simulink model "h01_MdeMgmt"  (R2024a)
settings: Solver=FixedStepDiscrete  StartTime=0.0  StopTime=mSim.dTime  FixedStep=mSim.dTime  MaxStep=0.0001  RelTol=0.0001
undefined symbols (not defined in the file): H01MDE, H01TRT
settings Model: Creator=admin  LastModifiedBy=admin
settings SolverCC: MaxConsecutiveZCs=10000  ZeroCrossAlgorithm=Adaptive  AlgebraicLoopSolver=TrustRegion
settings DataIOCC: SaveOutput=off  DSMLogging=off  InspectSignalLogs=on  SaveTime=off  SignalLoggingName=logsout_Validator
settings OptimizationCC: BlockReduction=off  DefaultParameterBehavior=Inlined  UseDivisionForNetSlopeComputation=UseDivisionForReciprocalsOfIntegersOnly  GainParamInheritBuiltInType=on  UseFloatMulNetSlope=on  DefaultUnderspecifiedDataType=single  InlineInvariantSignals=on  BitwiseOrLogicalOp=Logical operator  PassReuseOutputArgsAs=Individual arguments  EfficientFloat2IntCast=on  LifeSpan=Inf  OptimizeBlockOrder=speed  DifferentSizesBufferReuse=on  EfficientTunableParamExpr=on
settings DebuggingCC: SignalInfNanChecking=error  SignalRangeChecking=error  ReadBeforeWriteMsg=EnableAllAsError  WriteAfterWriteMsg=EnableAllAsError  WriteAfterReadMsg=EnableAllAsError  AlgebraicLoopMsg=error  ArtificialAlgebraicLoopMsg=error  SaveWithDisabledLinksMsg=error  SaveWithParameterizedLinksMsg=error  BlockPriorityViolationMsg=error  SolverPrmCheckMsg=error  InheritedTsInSrcMsg=error  SingleTaskRateTransMsg=error  TasksWithSamePriorityMsg=error  SigSpecEnsureSampleTimeMsg=error  CheckMatrixSingularityMsg=error  IntegerOverflowMsg=error  ParameterUnderflowMsg=error  ParameterPrecisionLossMsg=error  ParameterTunabilityLossMsg=error  UnderSpecifiedDataTypeMsg=error  UnnecessaryDatatypeConvMsg=warning  VectorMatrixConversionMsg=error  SignalLabelMismatchMsg=error  UnconnectedInputMsg=error  UnconnectedOutputMsg=error  UnconnectedLineMsg=error  SFcnCompatibilityMsg=error  UniqueDataStoreMsg=error  BusObjectLabelMismatch=error  RootOutportRequireBusObject=error  AssertControl=DisableAll  ModelReferenceIOMismatchMessage=error  UnknownTsInhSupMsg=error  ModelReferenceDataLoggingMessage=error  ModelReferenceSymbolNameMessage=none  StateNameClashWarn=warning  StrictBusMsg=ErrorOnBusTreatedAsVector  NonBusSignalsTreatedAsBus=error  SFInvalidInputDataAccessInChartInitDiag=error  SFTransitionOutsideNaturalParentDiag=error  SFUnreachableExecutionPathDiag=error  SFUndirectedBroadcastEventsDiag=error  SFTransitionActionBeforeConditionDiag=error  SFTemporalDelaySmallerThanSampleTimeDiag=error  SFSelfTransitionDiag=error  SFExecutionAtInitializationDiag=error  IntegerSaturationMsg=error  UnitsInconsistencyMsg=none  VariantConditionMismatch=error
settings HardwareCC: ProdBitPerPointer=32  ProdBitPerSizeT=32  ProdBitPerPtrDiffT=32  ProdLargestAtomicFloat=None  ProdWordSize=32  ProdLongLongMode=on  ProdHWDeviceType=Renesas->RH850
settings ModelReferenceCC: EnableRefExpFcnMdlSchedulingChecks=on  ModelReferenceNumInstancesAllowed=Single
settings SFSimCC: SimUseLocalCustomCode=off  CompileTimeRecursionLimit=0  EnableRuntimeRecursion=off  MATLABDynamicMemAlloc=off  CustomCodeUndefinedFunction=UseInterfaceOnly
settings RTWCC: Description=Embedded Coder  SystemTargetFile=ert.tlc  GenCodeOnly=on  TemplateMakefile=ert_default_tmf  GenerateReport=on  RTWUseLocalCustomCode=off  BuildConfiguration=Faster Runs  IncludeHyperlinkInReport=on  LaunchReport=on  GenerateTraceInfo=on  GenerateTraceReport=on  GenerateTraceReportSl=on  GenerateTraceReportSf=on  GenerateWebview=on  GenerateCodeMetricsReport=on  GenerateCodeReplacementReport=on  GPUComputeCapability=3.5  DLArmComputeVersion=19.05
settings RTWCC: CustomInclude=|
  | D:\1_Code\1_DWDC_CSPLUS_RH850\EX_EcompM24aBswR22\DWDCC_SW45CCLV_E2GHSM24A\TEMP
  | D:\1_Code\1_DWDC_CSPLUS_RH850\EX_EcompM24aBswR22\DWDCC_SW45CCLV_E2GHSM24A\ASW\eCompMbdCodeRlt\b01_OSnScheduler_ert_rtw
  | D:\1_Code\1_DWDC_CSPLUS_RH850\EX_EcompM24aBswR22\DWDCC_SW45CCLV_E2GHSM24A\ASW\eCompMbdCodeRlt\c01_MainAdc_ert_rtw
  | D:\1_Code\1_DWDC_CSPLUS_RH850\EX_EcompM24aBswR22\DWDCC_SW45CCLV_E2GHSM24A\ASW\eCompMbdCodeRlt\c02_SubAdc_ert_rtw
  | D:\1_Code\1_DWDC_CSPLUS_RH850\EX_EcompM24aBswR22\DWDCC_SW45CCLV_E2GHSM24A\ASW\eCompMbdCodeRlt\d01_Diaglnteg_ert_rtw
  | D:\1_Code\1_DWDC_CSPLUS_RH850\EX_EcompM24aBswR22\DWDCC_SW45CCLV_E2GHSM24A\ASW\eCompMbdCodeRlt\e01_MtrCtrl_VarGain_ert_rtw
  | D:\1_Code\1_DWDC_CSPLUS_RH850\EX_EcompM24aBswR22\DWDCC_SW45CCLV_E2GHSM24A\ASW\eCompMbdCodeRlt\e02_MtrCtrl_EstPst_ert_rtw
  | D:\1_Code\1_DWDC_CSPLUS_RH850\EX_EcompM24aBswR22\DWDCC_SW45CCLV_E2GHSM24A\ASW\eCompMbdCodeRlt\e03_MtrCtrl_MtrCtrl_ert_rtw
  | D:\1_Code\1_DWDC_CSPLUS_RH850\EX_EcompM24aBswR22\DWDCC_SW45CCLV_E2GHSM24A\ASW\eCompMbdCodeRlt\e04_MtrCtrl_PwmSet_ert_rtw
  | D:\1_Code\1_DWDC_CSPLUS_RH850\EX_EcompM24aBswR22\DWDCC_SW45CCLV_E2GHSM24A\ASW\eCompMbdCodeRlt\f01_CommRx1_ert_rtw
  | D:\1_Code\1_DWDC_CSPLUS_RH850\EX_EcompM24aBswR22\DWDCC_SW45CCLV_E2GHSM24A\ASW\eCompMbdCodeRlt\g01_CommTxDataSet1_ert_rtw
  | D:\1_Code\1_DWDC_CSPLUS_RH850\EX_EcompM24aBswR22\DWDCC_SW45CCLV_E2GHSM24A\ASW\eCompMbdCodeRlt\g02_CommTxDataSet2_ert_rtw
  | D:\1_Code\1_DWDC_CSPLUS_RH850\EX_EcompM24aBswR22\DWDCC_SW45CCLV_E2GHSM24A\ASW\eCompMbdCodeRlt\g03_CommTx_ert_rtw
  | D:\1_Code\1_DWDC_CSPLUS_RH850\EX_EcompM24aBswR22\DWDCC_SW45CCLV_E2GHSM24A\ASW\eCompMbdCodeRlt\h01_MdeMgmt_ert_rtw
  | D:\1_Code\1_DWDC_CSPLUS_RH850\EX_EcompM24aBswR22\DWDCC_SW45CCLV_E2GHSM24A\ASW\eCompMbdCodeRlt\i01_Dem_ert_rtw
  | D:\1_Code\1_DWDC_CSPLUS_RH850\EX_EcompM24aBswR22\DWDCC_SW45CCLV_E2GHSM24A\ASW\eCompMbdCodeRlt\j01_McuInit_ert_rtw
  | D:\1_Code\1_DWDC_CSPLUS_RH850\EX_EcompM24aBswR22\DWDCC_SW45CCLV_E2GHSM24A\ASW\eCompMbdCodeRlt\k01_NvM_ert_rtw
  | D:\1_Code\1_DWDC_CSPLUS_RH850\EX_EcompM24aBswR22\DWDCC_SW45CCLV_E2GHSM24A\ASW\eCompMbdCodeRlt\slprj\ert\_sharedutils
settings RTWCC: CustomInitializer=|
  | /* MISRA-C Dummy Code */
  | // H01STMDE.uDummy = 0U;
settings CodeAppCC: ForceParamTrailComments=on  IgnoreCustomStorageClasses=off  MATLABFcnDesc=on  MangleLength=4  CustomSymbolStrGlobalVar=GvH01$N$M  CustomSymbolStrType=StrH01$N$M  CustomSymbolStrFcn=$N$M$F  CustomSymbolStrMacro=$N$M  DefineNamingRule=UpperCase  ParamNamingRule=UpperCase  SimulinkBlockComments=off  EnableCustomComments=on  ReqsInCode=on
settings ERTTargetCC: UtilityFuncGeneration=Shared location  MultiwordLength=2048  IncludeMdlTerminateFcn=off  CombineSignalStateStructs=on  SuppressErrorStatus=on  SupportAbsoluteTime=off  SupportNonFinite=off  ParenthesesLevel=Maximum  CastingMode=Standards  GenerateSharedConstants=off  InlinedParameterPlacement=NonHierarchical  ERTSrcFileBannerTemplate=t_code_template.cgt  ERTHdrFileBannerTemplate=t_code_template.cgt  ERTDataSrcFileTemplate=t_code_template.cgt  ERTDataHdrFileTemplate=t_code_template.cgt  ERTCustomFileTemplate=example_file_process.tlc  ERTFilePackagingFormat=CompactWithDataFile  PreserveExpressionOrder=on  SuppressUnreachableDefaultCases=off  EnableSignedLeftShifts=off  EnableSignedRightShifts=off  IndentStyle=Allman  IndentSize=4
settings ConfigComp: CovSaveName=coveragedata  CovMetricSettings=we  CovEnableCumulative=off  CovSaveCumulativeToWorkspaceVar=on  CovSaveSingleToWorkspaceVar=on  CovOutputDir=sldv_output/$ModelName$\sldv_covoutput  PSModelRefIgnoreList=[]  PSEnableModelRefIgnoreList=off  PSModelRefMinMaxVerif=CheckAndConstrain  PSAutoStubLUT=on  DVTestSuiteOptimization=CombinedObjectives (Nonlinear Extended)  DVRebuildModelRepresentation=Always
settings SimscapeCC: SimscapeNormalizeSystem=off

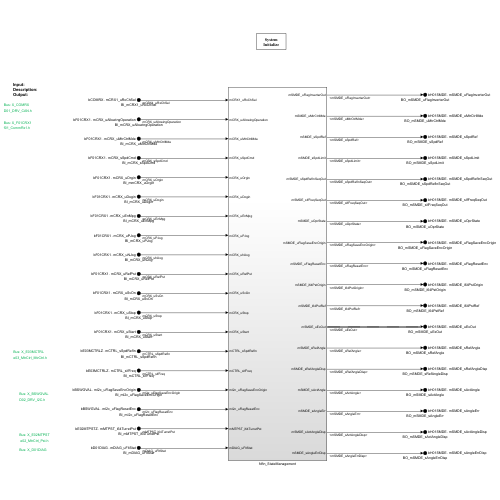
[thumbnail: Simulink's stored preview of the top-level diagram]
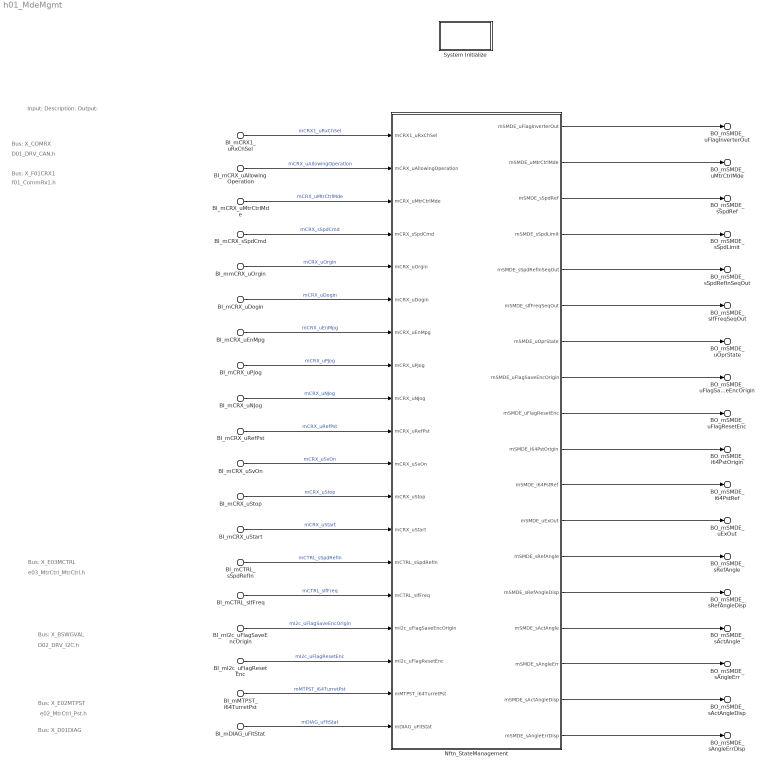
== system h01_MdeMgmt ==
  note: Bus: X_COMRX
  note: Bus: X_E03MCTRL
  note: e03_MtrCtrl_MtrCtrl.h
  note: D01_DRV_CAN.h
  note: Bus: X_BSWGVAL
  note: Bus: X_F01CRX1
  note: Input:
      | Description:
      | Output:
  note: Bus: X_E02MTPST
  note: e02_MtrCtrl_Pst.h
  note: D02_DRV_I2C.h
  note: f01_CommRx1.h
  note: Bus: X_D01DIAG
  BI_mCRX1_uRxChSel : Inport  Description=■ 설명: 운전 모드 설정 (0: I/O, 1: 통신)  PortName=bCOMRX  Element=mCRX1_uRxChSel
  BI_mCRX_uAllowingOperation : Inport  Description=■ 설명: 통신 모드 구동 신호 (0: 미구동, 1: 구동)  Port=2  PortName=bF01CRX1  Element=mCRX_uAllowingOperation
  BI_mCRX_uMtrCtrlMde : Inport  Description=■ 설명: 모터 구동 모드 (1_VF/2_V/4_CURR/8_TQ/16_SPD/32_PST/64_VALIGN/128_ALIGN/256_IF)  Port=2  PortName=bF01CRX1  Element=mCRX_uMtrCtrlMde
  BI_mCRX_uSvOn : Inport  Description=■ 설명: Digital Input Signal (서보 모터의 구동 신호, 0: 정지, 1: 구동)  Port=2  PortName=bF01CRX1  Element=mCRX_uSvOn
  BI_mCRX_uStart : Inport  Description=■ 설명: Digital Input Signal (구동 시작 신호, 상승 엣지 후 100msec 이상 검출 시 활성화)  Port=2  PortName=bF01CRX1  Element=mCRX_uStart
  BI_mCRX_uRefPst : Inport  Description=■ 설명: Digital Input Signal (위치 데이터 입력 신호 6Bit Binary Code)  Port=2  PortName=bF01CRX1  Element=mCRX_uRefPst
  BI_mCRX_uStop : Inport  Description=■ 설명: Digital Input Signal (동작 완료 신호)  Port=2  PortName=bF01CRX1  Element=mCRX_uStop
  BI_mmCRX_uOrgin : Inport  Description=■ 설명: Digital Input Signal (원점 설정 신호, 0: NA, 1: 원점 설정 활성화)  Port=2  PortName=bF01CRX1  Element=mCRX_uOrgin
  BI_mCRX_uDogin : Inport  Description=■ 설명: Digital Input Signal (원점 설정 초기화 신호, 0: NA, 1: 원점 초기화 활성화)  Port=2  PortName=bF01CRX1  Element=mCRX_uDogin
  BI_mCRX_uPJog : Inport  Description=■ 설명: Digital Input Signal (Manual CCW 구동 신호)  Port=2  PortName=bF01CRX1  Element=mCRX_uPJog
  BI_mCRX_uNJog : Inport  Description=■ 설명: Digital Input Signal (Manual CW 구동 신호)  Port=2  PortName=bF01CRX1  Element=mCRX_uNJog
  BI_mCRX_uEnMpg : Inport  Description=■ 설명: Digital Input Signal (미세 또는 단위 운전 설정, 0: 단위 운전, 1: 미세 운전)  Port=2  PortName=bF01CRX1  Element=mCRX_uEnMpg
  BI_mCRX_sSpdCmd : Inport  Description=■ 설명: 통신 모드 속도 지령  Port=2  PortName=bF01CRX1  Element=mCRX_sSpdCmd
  BI_mCTRL_sIfFreq : Inport  Description=■ 설명: IF Control Frequency  Port=3  PortName=bE03MCTRLZ  Element=mCTRL_sIfFreq
  BI_mCTRL_sSpdRefIn : Inport  Description=■ 설명: 속도 Slop 지령  Port=3  PortName=bE03MCTRLZ  Element=mCTRL_sSpdRefIn
  BI_mI2c_uFlagSaveEncOrigin : Inport  Description=■ 설명: 엔코더 원점 저장 활성화 신호  Port=4  PortName=bBSWGVAL  Element=mI2c_uFlagSaveEncOrigin
  BI_mI2c_uFlagResetEnc : Inport  Description=■ 설명: 엔코더 멀티턴 리셋 활성화 신호  Port=4  PortName=bBSWGVAL  Element=mI2c_uFlagResetEnc
  BI_mMTPST_i64TurretPst : Inport  Description=■ 설명: Turret Position  Port=5  PortName=bE02MTPSTZ  Element=mMTPST_i64TurretPst
  BI_mDIAG_uFltStat : Inport  Description=■ 설명: 고장 신호 대표 값  Port=6  PortName=bD01DIAG  Element=mDIAG_uFltStat
  Nftn_StateManagement : Subsystem
  System Initialize : Subsystem  mask(System Initialize){ShowInLibBrowser=0}
      mask prompts: ShowInLibBrowser "Simulink:masks:CustCodeMaskParam1_MP"
      settings: CopyFcn=cccopyfcn(gcb)  OpenFcn=ccopenfcn('System Initialize Function')
      mask Help: eval('feval(''rtwprivate'',''rtwhelpview'',''rtw_sys_initialize_block'')');
      mask DialogControl ShowInLibBrowser Prompt: 마스크 파라미터 1:
      mask Display: disp('System\nInitialize');
  BO_mSMDE_uFlagInverterOut : Outport  Description=■ 설명: Allow Operation 신호 (0: 구정 정지, 1: 구동)  PortName=bH01SMDE  Element=mSMDE_uFlagInverterOut
  BO_mSMDE_sSpdRefInSeqOut : Outport  Description=■ 설명: Speed Slop 제어를 위한 이전 지령 속도  PortName=bH01SMDE  Element=mSMDE_sSpdRefInSeqOut
  BO_mSMDE_sSpdLimit : Outport  Description=■ 설명: 속도 제한값  PortName=bH01SMDE  Element=mSMDE_sSpdLimit
  BO_mSMDE_sSpdRef : Outport  Description=■ 설명: 속도 지령  PortName=bH01SMDE  Element=mSMDE_sSpdRef
  BO_mSMDE_sIfFreqSeqOut : Outport  Description=■ 설명: 모터 구동 모드 (0_IO/1_VF/2_V/4_CURR/8_TQ/16_SPD/32_PST/64_VALIGN/128_ALIGN/256_IF)  PortName=bH01SMDE  Element=mSMDE_sIfFreqSeqOut
  BO_mSMDE_uMtrCtrlMde : Outport  Description=■ 설명: 운영 모드 (모터 구동 모드)  PortName=bH01SMDE  Element=mSMDE_uMtrCtrlMde
  BO_mSMDE_uOprState : Outport  Description=■ 설명: 운영 모드 (1H : Standby / 2H : JOG / 4H : MPG_JOG / 8H: Operating / 16H : Wait / 32H: Origin)  PortName=bH01SMDE  Element=mSMDE_uOprState
  BO_mSMDE_uFlagSaveEncOrigin : Outport  Description=■ 설명: 엔코더 원점 저장 활성화 신호  PortName=bH01SMDE  Element=mSMDE_uFlagSaveEncOrigin
  BO_mSMDE_uFlagResetEnc : Outport  Description=■ 설명: 엔코더 멀티턴 리셋 활성화 신호  PortName=bH01SMDE  Element=mSMDE_uFlagResetEnc
  BO_mSMDE_i64PstOrigin : Outport  Description=■ 설명: Encoder 원점 정보  PortName=bH01SMDE  Element=mSMDE_i64PstOrigin
  BO_mSMDE_i64PstRef : Outport  Description=■ 설명: Position Reference  PortName=bH01SMDE  Element=mSMDE_i64PstRef
  BO_mSMDE_sRefAngleDisp : Outport  Description=■ 설명: 터렛 지령 위치 모니터 값  PortName=bH01SMDE  Element=mSMDE_sRefAngleDisp
  BO_mSMDE_sActAngleDisp : Outport  Description=■ 설명: 터렛 지령 위치 모니터 값  PortName=bH01SMDE  Element=mSMDE_sActAngleDisp
  BO_mSMDE_sAngleErrDisp : Outport  Description="■ 설명: 터렛 현재 위치  오차 모니터 값"  PortName=bH01SMDE  Element=mSMDE_sAngleErrDisp
  BO_mSMDE_sRefAngle : Outport  Description=■ 설명: 터렛 지령 위치  PortName=bH01SMDE  Element=mSMDE_sRefAngle
  BO_mSMDE_sActAngle : Outport  Description=■ 설명: 터렛 현재 위치  PortName=bH01SMDE  Element=mSMDE_sActAngle
  BO_mSMDE_sAngleErr : Outport  Description=■ 설명: 터렛 위치 오차  PortName=bH01SMDE  Element=mSMDE_sAngleErr
  BO_mSMDE_uExOut : Outport  PortName=bH01SMDE  Element=mSMDE_uExOut
  wires:
  Nftn_StateManagement/8(mSMDE_uFlagSaveEncOrigin) -> BO_mSMDE_uFlagSaveEncOrigin/1
  Nftn_StateManagement/14(mSMDE_sRefAngleDisp) -> BO_mSMDE_sRefAngleDisp/1
  Nftn_StateManagement/17(mSMDE_sActAngleDisp) -> BO_mSMDE_sActAngleDisp/1
  BI_mCTRL_sIfFreq/1 -> Nftn_StateManagement/15(mCTRL_sIfFreq)  "mCTRL_sIfFreq"
  BI_mCRX_uMtrCtrlMde/1 -> Nftn_StateManagement/3(mCRX_uMtrCtrlMde)  "mCRX_uMtrCtrlMde"
  Nftn_StateManagement/18(mSMDE_sAngleErrDisp) -> BO_mSMDE_sAngleErrDisp/1
  BI_mCRX_uStop/1 -> Nftn_StateManagement/12(mCRX_uStop)  "mCRX_uStop"
  BI_mCRX_uSvOn/1 -> Nftn_StateManagement/11(mCRX_uSvOn)  "mCRX_uSvOn"
  BI_mCRX_uRefPst/1 -> Nftn_StateManagement/10(mCRX_uRefPst)  "mCRX_uRefPst"
  Nftn_StateManagement/7(mSMDE_uOprState) -> BO_mSMDE_uOprState/1
  Nftn_StateManagement/6(mSMDE_sIfFreqSeqOut) -> BO_mSMDE_sIfFreqSeqOut/1
  BI_mCRX_uNJog/1 -> Nftn_StateManagement/9(mCRX_uNJog)  "mCRX_uNJog"
  BI_mCRX_uAllowingOperation/1 -> Nftn_StateManagement/2(mCRX_uAllowingOperation)  "mCRX_uAllowingOperation"
  Nftn_StateManagement/16(mSMDE_sAngleErr) -> BO_mSMDE_sAngleErr/1
  BI_mCRX1_uRxChSel/1 -> Nftn_StateManagement/1(mCRX1_uRxChSel)  "mCRX1_uRxChSel"
  BI_mCRX_uStart/1 -> Nftn_StateManagement/13(mCRX_uStart)  "mCRX_uStart"
  Nftn_StateManagement/13(mSMDE_sRefAngle) -> BO_mSMDE_sRefAngle/1
  Nftn_StateManagement/15(mSMDE_sActAngle) -> BO_mSMDE_sActAngle/1
  BI_mCRX_sSpdCmd/1 -> Nftn_StateManagement/4(mCRX_sSpdCmd)  "mCRX_sSpdCmd"
  Nftn_StateManagement/1(mSMDE_uFlagInverterOut) -> BO_mSMDE_uFlagInverterOut/1
  BI_mCRX_uPJog/1 -> Nftn_StateManagement/8(mCRX_uPJog)  "mCRX_uPJog"
  Nftn_StateManagement/3(mSMDE_sSpdRef) -> BO_mSMDE_sSpdRef/1
  Nftn_StateManagement/5(mSMDE_sSpdRefInSeqOut) -> BO_mSMDE_sSpdRefInSeqOut/1
  BI_mI2c_uFlagResetEnc/1 -> Nftn_StateManagement/17(mI2c_uFlagResetEnc)  "mI2c_uFlagResetEnc"
  Nftn_StateManagement/9(mSMDE_uFlagResetEnc) -> BO_mSMDE_uFlagResetEnc/1
  Nftn_StateManagement/11(mSMDE_i64PstRef) -> BO_mSMDE_i64PstRef/1
  Nftn_StateManagement/10(mSMDE_i64PstOrigin) -> BO_mSMDE_i64PstOrigin/1
  BI_mCTRL_sSpdRefIn/1 -> Nftn_StateManagement/14(mCTRL_sSpdRefIn)  "mCTRL_sSpdRefIn"
  BI_mmCRX_uOrgin/1 -> Nftn_StateManagement/5(mCRX_uOrgin)  "mCRX_uOrgin"
  BI_mMTPST_i64TurretPst/1 -> Nftn_StateManagement/18(mMTPST_i64TurretPst)  "mMTPST_i64TurretPst"
  BI_mDIAG_uFltStat/1 -> Nftn_StateManagement/19(mDIAG_uFltStat)  "mDIAG_uFltStat"
  Nftn_StateManagement/2(mSMDE_uMtrCtrlMde) -> BO_mSMDE_uMtrCtrlMde/1
  BI_mCRX_uEnMpg/1 -> Nftn_StateManagement/7(mCRX_uEnMpg)  "mCRX_uEnMpg"
  Nftn_StateManagement/12(mSMDE_uExOut) -> BO_mSMDE_uExOut/1
  Nftn_StateManagement/4(mSMDE_sSpdLimit) -> BO_mSMDE_sSpdLimit/1
  BI_mCRX_uDogin/1 -> Nftn_StateManagement/6(mCRX_uDogin)  "mCRX_uDogin"
  BI_mI2c_uFlagSaveEncOrigin/1 -> Nftn_StateManagement/16(mI2c_uFlagSaveEncOrigin)  "mI2c_uFlagSaveEncOrigin"

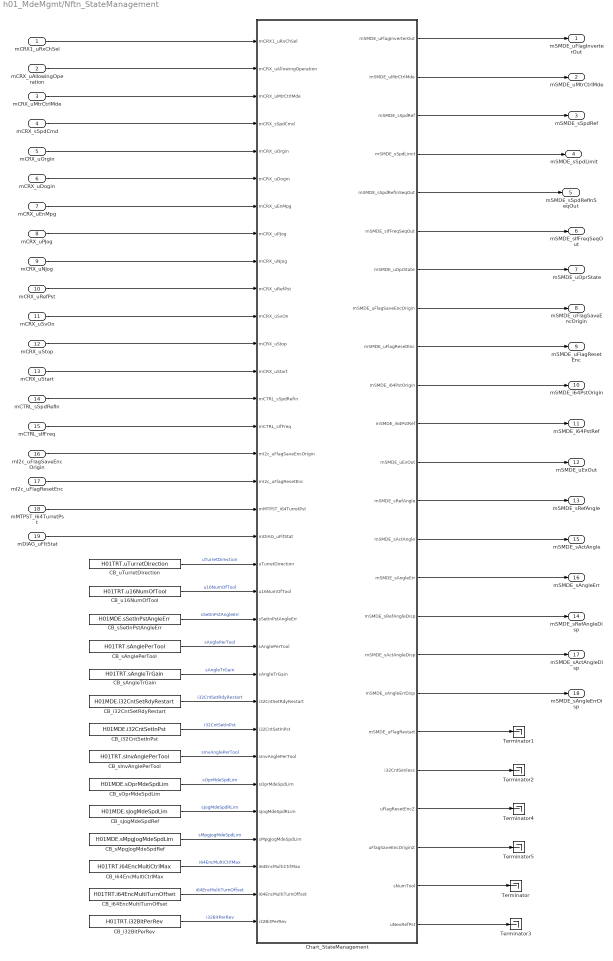
== system h01_MdeMgmt/Nftn_StateManagement ==
  mCRX1_uRxChSel : Inport
  mCRX_uAllowingOperation : Inport  Port=2
  mCRX_uMtrCtrlMde : Inport  Port=3
  mCRX_sSpdCmd : Inport  Port=4
  mCRX_uOrgin : Inport  Port=5
  mCRX_uDogin : Inport  Port=6
  mCRX_uEnMpg : Inport  Port=7
  mCRX_uPJog : Inport  Port=8
  mCRX_uNJog : Inport  Port=9
  mCRX_uRefPst : Inport  Port=10
  mCRX_uSvOn : Inport  Port=11
  mCRX_uStop : Inport  Port=12
  mCRX_uStart : Inport  Port=13
  mCTRL_sSpdRefIn : Inport  Port=14
  mCTRL_sIfFreq : Inport  Port=15
  mI2c_uFlagSaveEncOrigin : Inport  Port=16
  mI2c_uFlagResetEnc : Inport  Port=17
  mMTPST_i64TurretPst : Inport  Port=18
  mDIAG_uFltStat : Inport  Port=19
  CB_i32BitPerRev : Constant  Value=H01TRT.i32BitPerRev
  CB_i32CntSetInPst : Constant  Value=H01MDE.i32CntSetInPst
  CB_i32CntSetRdyRestart : Constant  Value=H01MDE.i32CntSetRdyRestart
  CB_i64EncMultiCtrlMax : Constant  Value=H01TRT.i64EncMultiCtrlMax
  CB_i64EncMultiTurnOffset : Constant  Value=H01TRT.i64EncMultiTurnOffset
  CB_sAnglePerTool : Constant  Value=H01TRT.sAnglePerTool
  CB_sAngleTrGain : Constant  Value=H01TRT.sAngleTrGain
  CB_sInvAnglePerTool : Constant  Value=H01TRT.sInvAnglePerTool
  CB_sJogMdeSpdRef : Constant  Value=H01MDE.sJogMdeSpdLim
  CB_sMpgJogMdeSpdRef : Constant  Value=H01MDE.sMpgJogMdeSpdLim
  CB_sOprMdeSpdLim : Constant  Value=H01MDE.sOprMdeSpdLim
  CB_sSetInPstAngleErr : Constant  Value=H01MDE.sSetInPstAngleErr
  CB_u16NumOfTool : Constant  Value=H01TRT.u16NumOfTool
  CB_uTurretDirection : Constant  Value=H01TRT.uTurretDirection
  Chart_StateManagement : Stateflow chart  TreatAsAtomicUnit=on
  Terminator{,1..5} (6 alike) : Terminator
  mSMDE_uFlagInverterOut : Outport
  mSMDE_uMtrCtrlMde : Outport  Port=2
  mSMDE_sSpdRef : Outport  Port=3
  mSMDE_sSpdLimit : Outport  Port=4
  mSMDE_sSpdRefInSeqOut : Outport  Port=5
  mSMDE_sIfFreqSeqOut : Outport  Port=6
  mSMDE_uOprState : Outport  Port=7
  mSMDE_uFlagSaveEncOrigin : Outport  Port=8
  mSMDE_uFlagResetEnc : Outport  Port=9
  mSMDE_i64PstOrigin : Outport  Port=10
  mSMDE_i64PstRef : Outport  Port=11
  mSMDE_uExOut : Outport  Port=12
  mSMDE_sRefAngle : Outport  Port=13
  mSMDE_sRefAngleDisp : Outport  Port=14
  mSMDE_sActAngle : Outport  Port=15
  mSMDE_sAngleErr : Outport  Port=16
  mSMDE_sActAngleDisp : Outport  Port=17
  mSMDE_sAngleErrDisp : Outport  Port=18
  wires:
  mCRX_uMtrCtrlMde/1 -> Chart_StateManagement/3(mCRX_uMtrCtrlMde)
  Chart_StateManagement/3(mSMDE_sSpdRef) -> mSMDE_sSpdRef/1
  Chart_StateManagement/5(mSMDE_sSpdRefInSeqOut) -> mSMDE_sSpdRefInSeqOut/1
  Chart_StateManagement/1(mSMDE_uFlagInverterOut) -> mSMDE_uFlagInverterOut/1
  mCRX_uAllowingOperation/1 -> Chart_StateManagement/2(mCRX_uAllowingOperation)
  Chart_StateManagement/6(mSMDE_sIfFreqSeqOut) -> mSMDE_sIfFreqSeqOut/1
  mCTRL_sSpdRefIn/1 -> Chart_StateManagement/14(mCTRL_sSpdRefIn)
  Chart_StateManagement/2(mSMDE_uMtrCtrlMde) -> mSMDE_uMtrCtrlMde/1
  mCTRL_sIfFreq/1 -> Chart_StateManagement/15(mCTRL_sIfFreq)
  mCRX_sSpdCmd/1 -> Chart_StateManagement/4(mCRX_sSpdCmd)
  mCRX1_uRxChSel/1 -> Chart_StateManagement/1(mCRX1_uRxChSel)
  Chart_StateManagement/7(mSMDE_uOprState) -> mSMDE_uOprState/1
  Chart_StateManagement/8(mSMDE_uFlagSaveEncOrigin) -> mSMDE_uFlagSaveEncOrigin/1
  Chart_StateManagement/10(mSMDE_i64PstOrigin) -> mSMDE_i64PstOrigin/1
  mCRX_uOrgin/1 -> Chart_StateManagement/5(mCRX_uOrgin)
  mCRX_uDogin/1 -> Chart_StateManagement/6(mCRX_uDogin)
  mI2c_uFlagSaveEncOrigin/1 -> Chart_StateManagement/16(mI2c_uFlagSaveEncOrigin)
  Chart_StateManagement/9(mSMDE_uFlagResetEnc) -> mSMDE_uFlagResetEnc/1
  mI2c_uFlagResetEnc/1 -> Chart_StateManagement/17(mI2c_uFlagResetEnc)
  Chart_StateManagement/11(mSMDE_i64PstRef) -> mSMDE_i64PstRef/1
  mCRX_uEnMpg/1 -> Chart_StateManagement/7(mCRX_uEnMpg)
  mCRX_uPJog/1 -> Chart_StateManagement/8(mCRX_uPJog)
  mCRX_uNJog/1 -> Chart_StateManagement/9(mCRX_uNJog)
  mMTPST_i64TurretPst/1 -> Chart_StateManagement/18(mMTPST_i64TurretPst)
  mCRX_uStart/1 -> Chart_StateManagement/13(mCRX_uStart)
  mCRX_uRefPst/1 -> Chart_StateManagement/10(mCRX_uRefPst)
  CB_sAnglePerTool/1 -> Chart_StateManagement/23(sAnglePerTool)  "sAnglePerTool"
  Chart_StateManagement/13(mSMDE_sRefAngle) -> mSMDE_sRefAngle/1
  CB_u16NumOfTool/1 -> Chart_StateManagement/21(u16NumOfTool)  "u16NumOfTool"
  Chart_StateManagement/12(mSMDE_uExOut) -> mSMDE_uExOut/1
  mDIAG_uFltStat/1 -> Chart_StateManagement/19(mDIAG_uFltStat)
  CB_i32CntSetRdyRestart/1 -> Chart_StateManagement/25(i32CntSetRdyRestart)  "i32CntSetRdyRestart"
  Chart_StateManagement/19(mSMDE_uFlagRestart) -> Terminator1/1
  Chart_StateManagement/20(i32CntSenless) -> Terminator2/1
  CB_sAngleTrGain/1 -> Chart_StateManagement/24(sAngleTrGain)  "sAngleTrGain"
  Chart_StateManagement/14(mSMDE_sActAngle) -> mSMDE_sActAngle/1
  Chart_StateManagement/21(uFlagResetEncZ) -> Terminator4/1
  Chart_StateManagement/22(uFlagSaveEncOriginZ) -> Terminator5/1
  mCRX_uSvOn/1 -> Chart_StateManagement/11(mCRX_uSvOn)
  CB_uTurretDirection/1 -> Chart_StateManagement/20(uTurretDirection)  "uTurretDirection"
  Chart_StateManagement/15(mSMDE_sAngleErr) -> mSMDE_sAngleErr/1
  CB_sSetInPstAngleErr/1 -> Chart_StateManagement/22(sSetInPstAngleErr)  "sSetInPstAngleErr"
  CB_i32CntSetInPst/1 -> Chart_StateManagement/26(i32CntSetInPst)  "i32CntSetInPst"
  mCRX_uStop/1 -> Chart_StateManagement/12(mCRX_uStop)
  CB_sInvAnglePerTool/1 -> Chart_StateManagement/27(sInvAnglePerTool)  "sInvAnglePerTool"
  CB_sJogMdeSpdRef/1 -> Chart_StateManagement/29(sJogMdeSpdRLim)  "sJogMdeSpdRLim"
  CB_sMpgJogMdeSpdRef/1 -> Chart_StateManagement/30(sMpgJogMdeSpdLim)  "sMpgJogMdeSpdLim"
  CB_i64EncMultiCtrlMax/1 -> Chart_StateManagement/31(i64EncMultiCtrlMax)  "i64EncMultiCtrlMax"
  CB_i64EncMultiTurnOffset/1 -> Chart_StateManagement/32(i64EncMultiTurnOffset)  "i64EncMultiTurnOffset"
  CB_i32BitPerRev/1 -> Chart_StateManagement/33(i32BitPerRev)  "i32BitPerRev"
  Chart_StateManagement/4(mSMDE_sSpdLimit) -> mSMDE_sSpdLimit/1
  CB_sOprMdeSpdLim/1 -> Chart_StateManagement/28(sOprMdeSpdLim)  "sOprMdeSpdLim"
  Chart_StateManagement/16(mSMDE_sRefAngleDisp) -> mSMDE_sRefAngleDisp/1
  Chart_StateManagement/18(mSMDE_sAngleErrDisp) -> mSMDE_sAngleErrDisp/1
  Chart_StateManagement/17(mSMDE_sActAngleDisp) -> mSMDE_sActAngleDisp/1
  Chart_StateManagement/23(sNumTool) -> Terminator/1
  Chart_StateManagement/24(uNexRefPst) -> Terminator3/1

== system h01_MdeMgmt/System Initialize ==

== stateflow chart h01_MdeMgmt/Nftn_StateManagement/Chart_StateManagement ==
  state Wait
    entry:
    mSMDE_uOprState = Cnst_OprMde16Wait;
    mSMDE_uFlagRestart = Cnst_u16False;
    i32CntSenless = 0;
    mSMDE_uExOut.uAlarm = Cnst_u16True;
    mSMDE_uExOut.uStadby = Cnst_u16False;
    during:
    Ftn_Wait();
    mSMDE_i64PstRef = mMTPST_i64TurretPst;
    state Ftn_Wait [function]
      (default) -> (junction 250) : {
          | mSMDE_uFlagInverterOut = Cnst_u16False;
          | }
      (junction 250) -> (junction 251) [order 1] : [i32CntSenless >= i32CntSetRdyRestart]
      (junction 250) -> (junction 252) [order 2] : {
          | i32CntSenless++;
          | }
      (junction 251) -> (junction 253) : {
          | i32CntSenless = i32CntSetRdyRestart;
          | mSMDE_uFlagRestart = Cnst_u16True;
          | }
      (junction 253) -> (junction 252)
      (junction 252) -> (junction 254)
  state Normal
    entry:
    mSMDE_uFlagRestart = Cnst_u16False;
    during:
    Ftn_CalActAngle();
    state Ftn_CalActAngle [function]
      (default) -> (junction 265) : // Calculation Acture Angle
      (junction 265) -> (junction 326) : {
          | sTemp = single(mMTPST_i64TurretPst - mSMDE_i64PstOrigin);
          | sTemp = sTemp * sAngleTrGain;
          | }
      (junction 326) -> (junction 328) [order 1] : [sTemp > Cnst_sZero]
      (junction 326) -> (junction 329) [order 2] : {
          | sTemp = (sTemp - single(int16(sTemp * Cnst_sInv360) * Cnst_s360)) + Cnst_s360;
          | }
      (junction 328) -> (junction 331) : {
          | sTemp = sTemp - single(int16(sTemp * Cnst_sInv360) * Cnst_s360);
          | }
      (junction 331) -> (junction 329)
      (junction 329) -> (junction 314)
      (junction 314) -> (junction 315) [order 1] : [sTemp < Cnst_sZero]
      (junction 314) -> (junction 319) [order 2]
      (junction 315) -> (junction 317) : {
          | sTemp = sTemp + Cnst_s360;
          | }
      (junction 319) -> (junction 321) [order 1] : [sTemp > Cnst_s360]
      (junction 319) -> (junction 316) [order 2] : {
          | sTemp = sTemp;
          | }
      (junction 321) -> (junction 322) : {
          | sTemp = sTemp - Cnst_s360;
          | }
      (junction 322) -> (junction 316)
      (junction 317) -> (junction 322)
      (junction 316) -> (junction 346)
      (junction 346) -> (junction 347) [order 1] : [uTurretDirection == Cnst_u16True]
      (junction 346) -> (junction 348) [order 2] : {
          | mSMDE_sActAngle = sTemp;
          | }
      (junction 347) -> (junction 349) : {
          | mSMDE_sActAngle = Cnst_s360 - sTemp;
          | }
      (junction 349) -> (junction 348)
      (junction 348) -> (junction 1542)
      (junction 1542) -> (junction 1543) [order 1] : [sRxRefAngle > Cnst_s360]
      (junction 1542) -> (junction 1560) [order 2]
      (junction 1543) -> (junction 1545) : {
          | mSMDE_sRefAngleDisp = sRxRefAngle - Cnst_s360;
          | }
      (junction 1560) -> (junction 1562) [order 1] : [sRxRefAngle < Cnst_sZero]
      (junction 1560) -> (junction 1544) [order 2] : {
          | mSMDE_sRefAngleDisp = sRxRefAngle;
          | }
      (junction 1562) -> (junction 1563) : {
          | mSMDE_sRefAngleDisp = sRxRefAngle + Cnst_s360;
          | }
      (junction 1563) -> (junction 1544)
      (junction 1545) -> (junction 1563)
      (junction 1544) -> (junction 1710)
      (junction 1710) -> (junction 1702) [order 1] : [mSMDE_sActAngle > Cnst_s360]
      (junction 1710) -> (junction 1696) [order 2]
      (junction 1702) -> (junction 1706) : {
          | mSMDE_sActAngleDisp = mSMDE_sActAngle - Cnst_s360;
          | }
      (junction 1696) -> (junction 1701) [order 1] : [mSMDE_sActAngle < Cnst_sZero]
      (junction 1696) -> (junction 1709) [order 2] : {
          | mSMDE_sActAngleDisp = mSMDE_sActAngle;
          | }
      (junction 1701) -> (junction 1708) : {
          | mSMDE_sActAngleDisp = mSMDE_sActAngle + Cnst_s360;
          | }
      (junction 1708) -> (junction 1709)
      (junction 1706) -> (junction 1708)
      (junction 1709) -> (junction 1678) : {
          | mSMDE_sAngleErrDisp = mSMDE_sRefAngleDisp - mSMDE_sActAngleDisp;
          | }
      (junction 1678) -> (junction 1682) [order 1] : [mSMDE_sAngleErrDisp > Cnst_s240]
      (junction 1678) -> (junction 1691) [order 2]
      (junction 1682) -> (junction 1684) : {
          | mSMDE_sAngleErrDisp = mSMDE_sAngleErrDisp - Cnst_s360;
          | }
      (junction 1691) -> (junction 1676) [order 1] : [mSMDE_sAngleErrDisp < -Cnst_s240]
      (junction 1691) -> (junction 1688) [order 2] : // No Action
      (junction 1676) -> (junction 1677) : {
          | mSMDE_sAngleErrDisp = mSMDE_sAngleErrDisp + Cnst_s360;
          | }
      (junction 1677) -> (junction 1688)
      (junction 1684) -> (junction 1677)
      (junction 1688) -> (junction 1713)
    note: 현재 위치 계산
    state Ftn_CalRefAngle [function]
      (default) -> (junction 799) : // Calculation Reference Angle
      (junction 799) -> (junction 896) [order 1] : [(mSMDE_i64PstOrigin ~= 0)&&(mCRX_uRefPst >= Cnst_u16One)]
      (junction 896) -> (junction 897)
      (junction 799) -> (junction 805) [order 2] : {
          | // Index 0 is not a valid value, but if index 0 is received, it is configured to move to the origin.
          | mSMDE_sRefAngle = Cnst_sZero;
          | }
      (junction 897) -> (junction 800) [order 1] : [(mCRX_uStart == Cnst_u16True)&&(uStartZ == Cnst_u16False)]
      (junction 897) -> (junction 900) [order 2] : // No Action
      (junction 800) -> (junction 801) : {
          | uFlagJogMde = Cnst_u16False;
          | }
      (junction 801) -> (junction 802) [order 1] : [mCRX_uRefPst > u16NumOfTool]
      (junction 801) -> (junction 803) [order 2] : {
          | uRefPst = mCRX_uRefPst;
          | }
      (junction 802) -> (junction 804) : {
          | uRefPst = u16NumOfTool;
          | }
      (junction 804) -> (junction 803)
      (junction 803) -> (junction 806) : {
          | sRxRefAngle = (single(uRefPst - Cnst_u16One) * sAnglePerTool);
          | Ftn_CalRefPst();
          | }
      (junction 806) -> (junction 900)
      (junction 900) -> (junction 805)
      (junction 805) -> (junction 807) : {
          | uStartZ = mCRX_uStart;
          | }
    note: Start 신호 입력시 Ref Angle 계산
    state Ftn_CalRefPst [function]
      (default) -> (junction 1433) : // Calculation Angle Error
      (junction 1433) -> (junction 1434) : {
          | mSMDE_uMtrCtrlMde = Cnst_MtrCtrlMde32Pst;
          | mSMDE_sAngleErr = sRxRefAngle - mSMDE_sActAngle;
          | }
      (junction 1434) -> (junction 1435) [order 1] : [mSMDE_sAngleErr < Cnst_sZero]
      (junction 1434) -> (junction 1436) [order 2] : {
          | sAbsAngleErr = mSMDE_sAngleErr;
          | }
      (junction 1435) -> (junction 1437) : {
          | sAbsAngleErr = -mSMDE_sAngleErr;
          | }
      (junction 1437) -> (junction 1436)
      (junction 1436) -> (junction 1438)
      (junction 1438) -> (junction 1439) [order 1] : // 각도 지령이 179~180도일 경우 또는 엔코더 포화시 근거리 운전 모드 -> 초기 멀티턴 방향으로 이동
          | [((sAbsAngleErr > Cnst_s179)&&(sAbsAngleErr < Cnst_s181))||((mSMDE_i64PstOrigin > i64EncMultiCtrlMax)&&(mSMDE_i64PstOrigin < (Cnst_i64EncMultiMax - i64EncMultiCtrlMax)))]
      (junction 1438) -> (junction 1440) [order 2]
      (junction 1439) -> (junction 1442)
      (junction 1440) -> (junction 1441) [order 1] : [mSMDE_sAngleErr > Cnst_s180]
      (junction 1442) -> (junction 1443) [order 1] : [uTurretDirection == Cnst_u16True]
      (junction 1440) -> (junction 1446) [order 2]
      (junction 1441) -> (junction 1467) : {
          | mSMDE_sRefAngle = mSMDE_sAngleErr - Cnst_s360;
          | }
      (junction 1442) -> (junction 1448) [order 2] : // uTurretDirection == Cnst_u16False
      (junction 1443) -> (junction 1444) : // uTurretDirection == Cnst_u16True
      (junction 1444) -> (junction 1445) [order 1] : [mSMDE_i64PstOrigin < i64EncMultiTurnOffset]
      (junction 1444) -> (junction 1450) [order 2] : // 멀티턴이 35535~65535 사이에 있을 경우 중앙(센터)에 가깝게 이동하기 위해 CW 방향으로 이동해야 함
      (junction 1445) -> (junction 1452) : // 멀티턴이 0~32768 사이에 있을 경우 중앙(센터)에 가깝게 이동하기 위해 CCW 방향으로 이동해야 함
      (junction 1446) -> (junction 1447) [order 1] : [mSMDE_sAngleErr < -Cnst_s180]
      (junction 1448) -> (junction 1449) [order 1] : [mSMDE_i64PstOrigin < i64EncMultiTurnOffset]
      (junction 1446) -> (junction 1465) [order 2] : {
          | mSMDE_sRefAngle = mSMDE_sAngleErr;
          | }
      (junction 1447) -> (junction 1466) : {
          | mSMDE_sRefAngle = mSMDE_sAngleErr + Cnst_s360;
          | }
      (junction 1448) -> (junction 1454) [order 2] : // 멀티턴이 35535~65535 사이에 있을 경우 중앙(센터)에 가깝게 이동하기 위해 CW 방향으로 이동해야 함
      (junction 1449) -> (junction 1456) : // 멀티턴이 0~32768 사이에 있을 경우 중앙(센터)에 가깝게 이동하기 위해 CCW 방향으로 이동해야 함
      (junction 1450) -> (junction 1451) [order 1] : [mSMDE_sAngleErr > Cnst_sZero]
      (junction 1452) -> (junction 1453) [order 1] : [mSMDE_sAngleErr > Cnst_sZero]
      (junction 1450) -> (junction 1464) [order 2] : {
          | // CCW 방향의 각도 지령일 경우  CCW 방향으로 이동(-180+360=180)
          | mSMDE_sRefAngle = mSMDE_sAngleErr;
          | }
      (junction 1451) -> (junction 1458) : {
          | // CW 방향의 각도 지령일 경우  CW 방향으로 이동(180=180)
          | mSMDE_sRefAngle = mSMDE_sAngleErr - Cnst_s360;
          | }
      (junction 1452) -> (junction 1459) [order 2] : {
          | // CCW 방향의 각도 지령일 경우  CCW 방향으로 이동(-180=-180)
          | mSMDE_sRefAngle = mSMDE_sAngleErr + Cnst_s360;
          | }
      (junction 1453) -> (junction 1460) : {
          | // CW 방향의 각도 지령일 경우  CCW 방향으로 이동(180-360=-180)
          | mSMDE_sRefAngle = mSMDE_sAngleErr;
          | }
      (junction 1454) -> (junction 1455) [order 1] : [mSMDE_sAngleErr > Cnst_sZero]
      (junction 1456) -> (junction 1457) [order 1] : [mSMDE_sAngleErr > Cnst_sZero]
      (junction 1454) -> (junction 1468) [order 2] : {
          | // CCW 방향의 각도 지령일 경우  CCW 방향으로 이동(-180+360=180)
          | mSMDE_sRefAngle = mSMDE_sAngleErr + Cnst_s360;
          | }
      (junction 1455) -> (junction 1461) : {
          | // CW 방향의 각도 지령일 경우  CW 방향으로 이동(180=180)
          | mSMDE_sRefAngle = mSMDE_sAngleErr;
          | }
      (junction 1456) -> (junction 1462) [order 2] : {
          | // CCW 방향의 각도 지령일 경우  CCW 방향으로 이동(-180=-180)
          | mSMDE_sRefAngle = mSMDE_sAngleErr;
          | }
      (junction 1457) -> (junction 1463) : {
          | // CW 방향의 각도 지령일 경우  CCW 방향으로 이동(180-360=-180)
          | mSMDE_sRefAngle = mSMDE_sAngleErr - Cnst_s360;
          | }
      (junction 1459) -> (junction 1458)
      (junction 1460) -> (junction 1459)
      (junction 1458) -> (junction 1464)
      (junction 1462) -> (junction 1461)
      (junction 1463) -> (junction 1462)
      (junction 1464) -> (junction 1463)
      (junction 1461) -> (junction 1468)
      (junction 1466) -> (junction 1465)
      (junction 1467) -> (junction 1466)
      (junction 1468) -> (junction 1467)
      (junction 1465) -> (junction 1469)
      (junction 1469) -> (junction 1470) [order 1] : [uTurretDirection == Cnst_u16True]
      (junction 1469) -> (junction 1471) [order 2] : {
          | mSMDE_i64PstRef = mMTPST_i64TurretPst + int64(single(i32BitPerRev) * (mSMDE_sRefAngle * Cnst_sInv360));
          | }
      (junction 1470) -> (junction 1472) : {
          | mSMDE_i64PstRef = mMTPST_i64TurretPst - int64(single(i32BitPerRev) * (mSMDE_sRefAngle * Cnst_sInv360));
          | }
      (junction 1472) -> (junction 1471)
      (junction 1471) -> (junction 1473)
    note: Ref Angle 재 계산 (가까운 목표 위치)
    note: // mSMDE_i64PstRef 초기값 설정할 것
    state Ftn_CalExOutPst [function]
      note: uNumTool = (Deg / sAnglePerTool) + 1 +0.05;  // 소수 2째자리 반올림 0.05 반영
          | uNumTool = (Deg * sInvAnglePerTool) + 1 +0.05;
          | uNumTool = ((Deg * sInvAnglePerTool) + 1 +0.05) * 10;    // x10
          | uNumTool = single(int16(((Deg * sInvAnglePerTool) + 1 +0.05) * 10)) * 0.1;    // 소숫점이하 버림
          |
          | if(int16(uNumTool) == uNumTool)           // 정수 구하기
          | {
          | 	out = uint16(uNumTool);
          | }
      note: ▶ 현재 위치를 외부 24 V 신호로 출력
      (default) -> (junction 820) : // Calculating the Current Position and Setting the Digital Output
      (junction 820) -> (junction 821) : {
          | sNumTool = single(int16(((mSMDE_sActAngle * sInvAnglePerTool) + 1.0 + 0.05) * 10)) * 0.1;    // 소숫점이하 버림
          | }
      (junction 821) -> (junction 822) [order 1] : [mSMDE_sActAngle > (Cnst_s360 - sSetInPstAngleErr)]
      (junction 821) -> (junction 823) [order 2]
      (junction 822) -> (junction 825) : {
          | mSMDE_uExOut.uActPst = Cnst_u16One;
          | }
      (junction 823) -> (junction 824) [order 1] : [single(int16(sNumTool)*10.0) == (sNumTool*10.0)]
      (junction 823) -> (junction 826) [order 2] : {
          | mSMDE_uExOut.uActPst = Cnst_u16Zero;
          | }
      (junction 824) -> (junction 827) : {
          | mSMDE_uExOut.uActPst = uint16(sNumTool);
          | }
      (junction 825) -> (junction 827)
      (junction 827) -> (junction 826)
      (junction 826) -> (junction 828)
    state Standby
      entry:
      mSMDE_uOprState = Cnst_OprMde1Standby;
      uFlagCmpltOpMde = Cnst_u16False;
      mSMDE_uExOut.uAlarm = Cnst_u16False;
      mSMDE_uExOut.uStadby = Cnst_u16True;
      // mSMDE_i64PstRef = mMTPST_i64TurretPst;
      mSMDE_sSpdLimit = sOprMdeSpdLim;
      during:
      Ftn_Standby();
      Ftn_CalExOutPst();
      state Ftn_Standby [function]
        note: CAN 통신을 이용한 제어
            | ▷ 일반 모드
            |    -. mCRX_uCtrlMde0Digt1Can = 1
            |    -. mCRX_uSvOn = 0
            |
            | ▷ 위치 제어 모드
            |    -. mCRX_uCtrlMde0Digt1Can = 1
            |    -. mCRX_uSvOn = 1
            |
            | mCRX_uSvOn 이 활성화된 경우 위치제어 모드로 운전함
        (default) -> (junction 62) : // Operation mode set (0: I/O, 1: Communication)
        (junction 62) -> (junction 65) [order 1] : [mCRX1_uRxChSel == Cnst_u16True]
        (junction 62) -> (junction 1731) [order 2] : // I/O Operation
        (junction 65) -> (junction 1742) : // Communication
        (junction 1731) -> (junction 1745) [order 1] : [mCRX_uSvOn == Cnst_u16True]
        (junction 1731) -> (junction 61) [order 2] : {
            | mSMDE_uFlagInverterOut = Cnst_u16False;
            | mSMDE_uMtrCtrlMde = Cnst_u16Zero;
            | mSMDE_sSpdRef = Cnst_sZero;
            | mSMDE_i64PstRef = mMTPST_i64TurretPst;
            | }
        (junction 1745) -> (junction 1749) : {
            | mSMDE_uFlagInverterOut = Cnst_u16True;
            | mSMDE_uMtrCtrlMde = Cnst_MtrCtrlMde32Pst;
            | }
        (junction 1742) -> (junction 1733) [order 1] : [mCRX_uSvOn == Cnst_u16True]
        (junction 1742) -> (junction 63) [order 2] : {
            | // CAN Operation
            | mSMDE_uFlagInverterOut = mCRX_uAllowingOperation;
            | mSMDE_uMtrCtrlMde = mCRX_uMtrCtrlMde;
            | mSMDE_sSpdRef = mCRX_sSpdCmd;
            | }
        (junction 1733) -> (junction 1734) : {
            | mSMDE_uFlagInverterOut = Cnst_u16True;
            | mSMDE_uMtrCtrlMde = Cnst_MtrCtrlMde32Pst;
            | }
        (junction 1749) -> (junction 61)
        (junction 63) -> (junction 1749)
        (junction 1734) -> (junction 63)
        (junction 61) -> (junction 64) : {
            | mSMDE_sSpdRefInSeqOut = mCTRL_sSpdRefIn;
            | mSMDE_sIfFreqSeqOut = mCTRL_sIfFreq;
            | uOrginZ = mCRX_uOrgin;
            | uDoginZ = mCRX_uDogin;
            | uFlagResetEncZ = mI2c_uFlagResetEnc;
            | uFlagSaveEncOriginZ = mI2c_uFlagSaveEncOrigin;
            | }
    state OriginDogin
      entry:
      mSMDE_uOprState = Cnst_OprMde32Origin;
      during:
      Ftn_OriginDogin();
      exit:
      mSMDE_uFlagSaveEncOrigin = Cnst_u16False;
      state Ftn_OriginDogin [function]
        (default) -> (junction 299) : {
            | mSMDE_uFlagInverterOut = Cnst_u16False;
            | }
        (junction 299) -> (junction 301) [order 1] : [(mCRX_uOrgin == Cnst_u16True)&&(mCRX_uDogin == Cnst_u16True)]
        (junction 299) -> (junction 96) [order 2]
        (junction 301) -> (junction 303) : // No Action
        (junction 96) -> (junction 115) [order 1] : [mCRX_uOrgin == Cnst_u16True]
        (junction 96) -> (junction 291) [order 2]
        (junction 115) -> (junction 112) : {
            | // Act uOrigin
            | mSMDE_uFlagSaveEncOrigin = Cnst_u16True;
            | mSMDE_sRefAngle = Cnst_sZero;
            | mSMDE_i64PstOrigin = mMTPST_i64TurretPst;
            | mSMDE_uExOut.uOrgNotDef = Cnst_u16False;
            | mSMDE_uExOut.uInPst = Cnst_u16True;
            | }
        (junction 291) -> (junction 293) [order 1] : [mCRX_uDogin == Cnst_u16True]
        (junction 291) -> (junction 117) [order 2] : // No Action
        (junction 293) -> (junction 294) : {
            | // Act uDogin
            | mSMDE_uFlagResetEnc = Cnst_u16True;
            | mSMDE_i64PstOrigin = 0;
            | mSMDE_uExOut.uOrgNotDef = Cnst_u16True;
            | }
        (junction 294) -> (junction 117)
        (junction 112) -> (junction 294)
        (junction 303) -> (junction 112)
        (junction 117) -> (junction 118) : {
            | mSMDE_i64PstRef = 0;
            | uOrginZ = mCRX_uOrgin;
            | uDoginZ = mCRX_uDogin;
            | uFlagResetEncZ = mI2c_uFlagResetEnc;
            | uFlagSaveEncOriginZ = mI2c_uFlagSaveEncOrigin;
            | mSMDE_i64PstRef = mMTPST_i64TurretPst;
            | }
    state MpgJOG
      entry:
      mSMDE_uOprState = Cnst_OprMde4Mpg;
      during:
      mSMDE_uFlagInverterOut = mCRX_uSvOn;
      Ftn_CalExOutPst();
      Ftn_MpgJogMde();
      state Ftn_MpgJogMde [function]
        (default) -> (junction 136)
        (junction 136) -> (junction 137) [order 1] : [(mCRX_uPJog == Cnst_u16True)&&(mCRX_uNJog == Cnst_u16True)]
        (junction 136) -> (junction 841) [order 2]
        (junction 137) -> (junction 139) : {
            | mSMDE_uMtrCtrlMde = Cnst_MtrCtrlMde32Pst;
            | mSMDE_sSpdRef = Cnst_sZero;
            | }
        (junction 841) -> (junction 843) [order 1] : [mCRX_uPJog == Cnst_u16True]
        (junction 841) -> (junction 1088) [order 2]
        (junction 843) -> (junction 844) : {
            | mSMDE_uMtrCtrlMde = Cnst_MtrCtrlMde16Spd;
            | mSMDE_sSpdRef = sMpgJogMdeSpdLim;
            | }
        (junction 1088) -> (junction 1090) [order 1] : [mCRX_uNJog == Cnst_u16True]
        (junction 1088) -> (junction 138) [order 2] : {
            | mSMDE_uMtrCtrlMde = Cnst_MtrCtrlMde32Pst;
            | mSMDE_sSpdRef = Cnst_sZero;
            | }
        (junction 1090) -> (junction 1091) : {
            | mSMDE_uMtrCtrlMde = Cnst_MtrCtrlMde16Spd;
            | mSMDE_sSpdRef = -sMpgJogMdeSpdLim;
            | }
        (junction 1091) -> (junction 138)
        (junction 844) -> (junction 1091)
        (junction 139) -> (junction 844)
        (junction 138) -> (junction 857) : {
            | mSMDE_i64PstRef = mMTPST_i64TurretPst;
            | }
    state OperNJog
      entry:
      i32CntSenless = 0;
      during:
      mSMDE_uFlagInverterOut = mCRX_uSvOn;
      Ftn_MoveToRefPst();
      Ftn_CalAngleError();
      Ftn_CalExOutPst();
      state Ftn_MoveToRefPst [function]
        (default) -> (junction 1097)
        (junction 1097) -> (junction 1098) [order 1] : [((mCRX_uPJog == Cnst_u16True)&&(mCRX_uNJog == Cnst_u16True))||((mCRX_uPJog == Cnst_u16False)&&(mCRX_uNJog == Cnst_u16False))]
        (junction 1098) -> (junction 1101) : {
            | mSMDE_uOprState = Cnst_OprMde8Operation;
            | mSMDE_uMtrCtrlMde = Cnst_MtrCtrlMde32Pst;
            | }
        (junction 1097) -> (junction 1099) [order 2] : // Activation Jog Mode
            | {
            | mSMDE_uOprState = Cnst_OprMde2Jog;
            | mSMDE_uMtrCtrlMde = Cnst_MtrCtrlMde16Spd;
            | uFlagStepJogMde = Cnst_u16True;
            | uFlagJogMde = Cnst_u16True;
            | }
        (junction 1099) -> (junction 1100) [order 1] : [mCRX_uPJog == Cnst_u16True]
        (junction 1100) -> (junction 1105)
        (junction 1099) -> (junction 1103) [order 2]
        (junction 1105) -> (junction 1106) [order 1] : [uFalg_NJog_Step == Cnst_u16False]
        (junction 1103) -> (junction 1104) [order 1] : [uFalg_PJog_Step == Cnst_u16False]
        (junction 1104) -> (junction 1428) : {
            | // uFalg_NJog_Step = Cnst_u16True;;
            | }
        (junction 1105) -> (junction 1114) [order 2] : // No Action
        (junction 1106) -> (junction 1154) : {
            | // uFalg_PJog_Step = Cnst_u16True;
            | }
        (junction 1103) -> (junction 1112) [order 2] : // No Action
        (junction 1101) -> (junction 1102) [order 1] : [uFlagStepJogMde == Cnst_u16True]
        (junction 1101) -> (junction 1533) [order 2] : {
            | mSMDE_sSpdLimit = sOprMdeSpdLim;
            | }
        (junction 1102) -> (junction 1118) : {
            | mSMDE_sSpdLimit = sJogMdeSpdRLim;
            | }
        (junction 1428) -> (junction 1421) [order 1] : [uTurretDirection == Cnst_u16True]
        (junction 1154) -> (junction 1156) [order 1] : [uTurretDirection == Cnst_u16True]
        (junction 1428) -> (junction 1422) [order 2] : {
            | mSMDE_sSpdRef = -sJogMdeSpdRLim
            | uNexRefPst = uint16(sNumTool - Cnst_sOneHalf);
            | }
        (junction 1421) -> (junction 1426) : {
            | mSMDE_sSpdRef = sJogMdeSpdRLim
            | uNexRefPst = uint16(sNumTool + Cnst_sHalf);
            | }
        (junction 1154) -> (junction 1111) [order 2] : {
            | mSMDE_sSpdRef = sJogMdeSpdRLim;
            | uNexRefPst = uint16(sNumTool + Cnst_sHalf);
            | }
        (junction 1156) -> (junction 1157) : {
            | mSMDE_sSpdRef = -sJogMdeSpdRLim;
            | uNexRefPst = uint16(sNumTool - Cnst_sOneHalf);
            | }
        (junction 1118) -> (junction 1533)
        (junction 1422) -> (junction 1112)
        (junction 1426) -> (junction 1422)
        (junction 1114) -> (junction 1426)
        (junction 1111) -> (junction 1114)
        (junction 1157) -> (junction 1111)
        (junction 1533) -> (junction 1115) : {
            | Ftn_CalRefAngle();
            | }
        (junction 1112) -> (junction 1715) : {
            | mSMDE_sRefAngle = (single(uNexRefPst) * sAnglePerTool);
            | mSMDE_sAngleErr = (mSMDE_sRefAngle - mSMDE_sActAngleDisp);
            | mSMDE_i64PstRef = mMTPST_i64TurretPst + int64(single(i32BitPerRev) * (mSMDE_sAngleErr * Cnst_sInv360));
            | }
        (junction 1115) -> (junction 1715)
        (junction 1715) -> (junction 1119)
      state Ftn_CalAngleError [function]
        (default) -> (junction 761) : // Calculation Angle Error
        (junction 761) -> (junction 1554) : {
            | //mSMDE_uMtrCtrlMde = Cnst_MtrCtrlMde32Pst;
            | mSMDE_sAngleErr = mSMDE_sRefAngle - mSMDE_sActAngle;
            | }
        (junction 1554) -> (junction 1555) [order 1] : [mSMDE_sAngleErr > Cnst_s360]
        (junction 1554) -> (junction 1649) [order 2] : // No Action
        (junction 1555) -> (junction 1557) : {
            | mSMDE_sAngleErr = mSMDE_sAngleErr - Cnst_s360;
            | }
        (junction 1649) -> (junction 1651) [order 1] : [mSMDE_sAngleErr < -Cnst_sZero]
        (junction 1649) -> (junction 1556) [order 2] : {
            | mSMDE_sAngleErr = mSMDE_sAngleErr;
            | }
        (junction 1651) -> (junction 1652) : {
            | mSMDE_sAngleErr = mSMDE_sAngleErr + Cnst_s360;
            | }
        (junction 1652) -> (junction 1556)
        (junction 1557) -> (junction 1652)
        (junction 1556) -> (junction 762)
        (junction 762) -> (junction 763) [order 1] : [mSMDE_sAngleErrDisp < Cnst_sZero]
        (junction 762) -> (junction 764) [order 2] : {
            | sAbsAngleErr = mSMDE_sAngleErrDisp;
            | }
        (junction 763) -> (junction 765) : {
            | sAbsAngleErr = -mSMDE_sAngleErrDisp;
            | }
        (junction 765) -> (junction 764)
        (junction 764) -> (junction 766)
        (junction 766) -> (junction 767) [order 1] : [(sAbsAngleErr < sSetInPstAngleErr)||(sAbsAngleErr > (Cnst_s360 - sSetInPstAngleErr))]
        (junction 766) -> (junction 772) [order 2] : {
            | mSMDE_uExOut.uInPst = Cnst_u16False;
            | i32CntSenless = 0;
            | }
        (junction 767) -> (junction 768)
        (junction 768) -> (junction 769) [order 1] : [i32CntSenless >= i32CntSetInPst]
        (junction 768) -> (junction 773) [order 2] : {
            | i32CntSenless++;
            | }
        (junction 769) -> (junction 774) : {
            | i32CntSenless = i32CntSetInPst;
            | mSMDE_uExOut.uInPst = Cnst_u16True;
            | uFlagStepJogMde = Cnst_u16False;
            | uFalg_PJog_Step = Cnst_u16False;
            | uFalg_NJog_Step = Cnst_u16False;
            | uFlagCmpltOpMde = Cnst_u16True;
            | }
        (junction 773) -> (junction 772)
        (junction 774) -> (junction 773)
        (junction 1727) -> (junction 1728) [commented out] : [mCRX_uStop == Cnst_u16True]
        (junction 772) -> (junction 776)
        (junction 1727) -> (junction 1730) [commented out] : // No Action
        (junction 1728) -> (junction 1729) [commented out] : {
            | mSMDE_uFlagInverterOut = Cnst_u16False;
            | i32CntSenless = 0;
            | }
        (junction 1729) -> (junction 1730) [commented out]
    (default) -> Standby
    Standby -> OriginDogin [order 1] : [((mCRX_uOrgin == Cnst_u16True)&&(uOrginZ == Cnst_u16False))||((mCRX_uDogin == Cnst_u16True)&&(uDoginZ == Cnst_u16False))]
    OriginDogin -> Standby [order 1] : [(mI2c_uFlagResetEnc == Cnst_u16False)&&(uFlagResetEncZ == Cnst_u16True)]
    OriginDogin -> Standby [order 2] : [(mI2c_uFlagSaveEncOrigin == Cnst_u16False)&&(uFlagSaveEncOriginZ == Cnst_u16True)]
    Standby -> MpgJOG [order 2] : [(mCRX_uSvOn == Cnst_u16True)&&(mCRX_uEnMpg == Cnst_u16True)]
    MpgJOG -> Standby : [(mCRX_uSvOn == Cnst_u16False)||(mCRX_uEnMpg == Cnst_u16False)]
    OperNJog -> MpgJOG [order 2] : [(mCRX_uSvOn == Cnst_u16True)&&(mCRX_uEnMpg == Cnst_u16True)]
    Standby -> OperNJog [order 3] : [(mCRX_uSvOn == Cnst_u16True)&&(mSMDE_i64PstOrigin ~= 0)&&((mCRX_uPJog == Cnst_u16True)||(mCRX_uNJog == Cnst_u16True))]
    Standby -> OperNJog [order 4] : [(mCRX_uSvOn == Cnst_u16True)&&(mSMDE_i64PstOrigin ~= 0)&&(mCRX_uStart == Cnst_u16True)&&(uStartZ == Cnst_u16False)]
    OperNJog -> Standby [order 1] : [(mCRX_uSvOn == Cnst_u16False)||(uFlagCmpltOpMde == Cnst_u16True)]
  note: Cnst_OprMde1Standby
      | Cnst_OprMde2Jog
      | Cnst_OprMde4Mpg
      | Cnst_OprMde8Operation
      | Cnst_OprMde16Wait
  (default) -> Normal
  Normal -> Wait : [mDIAG_uFltStat == Cnst_u16True]
  Wait -> Normal : [(mDIAG_uFltStat == Cnst_u16False)&&(mSMDE_uFlagRestart == Cnst_u16True)]
  data: mCRX1_uRxChSel input; mCRX_uAllowingOperation input; mCRX_uMtrCtrlMde input; mCRX_sSpdCmd input; mCRX_uOrgin input; mCRX_uDogin input; mCRX_uEnMpg input; mCRX_uPJog input; mCRX_uNJog input; mCRX_uRefPst input; mCRX_uSvOn input; mCRX_uStop input; mCRX_uStart input; mCTRL_sSpdRefIn input; mCTRL_sIfFreq input; mSMDE_uFlagInverterOut output uint16; mSMDE_uMtrCtrlMde output uint16; mSMDE_sSpdRef output single; mSMDE_sSpdLimit output single; mSMDE_sSpdRefInSeqOut output single; mSMDE_sIfFreqSeqOut output single; Cnst_u16False constant uint16 =CnstNr.C_u16_0; Cnst_u16Zero constant uint16 =CnstNr.C_u16_0; Cnst_sZero constant single =CnstNr.C_sZero; mSMDE_uOprState output uint16; mSMDE_uFlagSaveEncOrigin output uint16; mSMDE_uFlagResetEnc output uint16; mSMDE_i64PstOrigin output int64 =4294180863; Cnst_OprMde1Standby constant uint16 =1; Cnst_OprMde32Origin constant uint16 =32; Cnst_u16True constant uint16 =CnstNr.C_u16_1; mI2c_uFlagSaveEncOrigin input; mI2c_uFlagResetEnc input; mSMDE_i64PstRef output int64; mSMDE_uExOut output Bus: X_H01EXO; Cnst_OprMde4Mpg constant uint16 =4; mMTPST_i64TurretPst input; mDIAG_uFltStat input; uTurretDirection input; u16NumOfTool input; sSetInPstAngleErr input; mSMDE_sRefAngle output single; mSMDE_sActAngle output single; mSMDE_sAngleErr output single; mSMDE_sRefAngleDisp output single; mSMDE_sActAngleDisp output single; mSMDE_sAngleErrDisp output single; sAnglePerTool input; sAngleTrGain input; Cnst_u16One constant uint16 =CnstNr.C_u16_1; uRefPst local uint16; Cnst_OprMde16Wait constant uint16 =16; mSMDE_uFlagRestart output uint16; i32CntSenless output int32; i32CntSetRdyRestart input; uDoginZ local uint16; uOrginZ local uint16; uFlagResetEncZ output uint16; uFlagSaveEncOriginZ output uint16; Cnst_s360 constant single =360; Cnst_sInv360 constant single =1/360; sTemp local single; Cnst_OprMde8Operation constant uint16 =8; sAbsAngleErr local single; i32CntSetInPst input; sInvAnglePerTool input; sOprMdeSpdLim input; uFlagCmpltOpMde local uint16; Cnst_MtrCtrlMde16Spd constant uint16 =CnstMde.C_MODE16_SPD; sJogMdeSpdRLim input; Cnst_MtrCtrlMde32Pst constant uint16 =CnstMde.C_MODE32_PST; Cnst_OprMde2Jog constant uint16 =2; sMpgJogMdeSpdLim input; uFalg_NJog_Step local uint16; uFalg_PJog_Step local uint16; Cnst_s179 constant single =179; Cnst_s181 constant single =181; i64EncMultiCtrlMax input; Cnst_i64EncMultiMax constant int64 =65535; i64EncMultiTurnOffset input; Cnst_s180 constant single =180; i32BitPerRev input; uFlagJogMde local uint16; uFlagStepJogMde local uint16; Cnst_sHalf constant single =0.5; uStartZ local uint16; Cnst_s240 constant single =240; sRxRefAngle local single; sNumTool output single; uNexRefPst output uint16; Cnst_sOneHalf constant single =1.5
